simulink model "e1516sim"  (R2022a)
settings: Solver=VariableStepAuto  StartTime=0.0  StopTime=10  RelTol=1e-3
values from neighbouring files (symbols this model uses):
  delta_a = 0    [e1516.m]    (also in l6.m)
  dt = 0    [e1516.m]
  dy = 0    [e1516.m]
  rho = 1    [e1516.m]    (also in l6.m = 0)
libraries: cstblocks x2, simulink x1
settings Model: Creator=apple  LastModifiedBy=apple

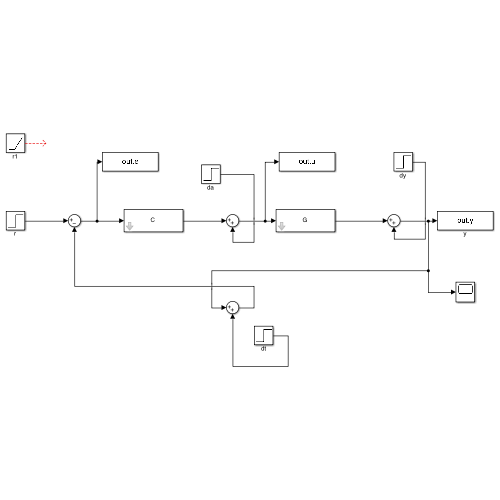
[thumbnail: Simulink's stored preview of the top-level diagram]
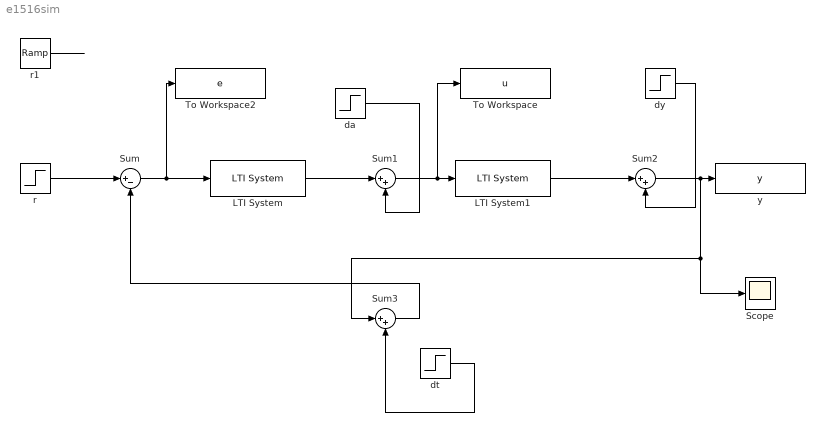
== system e1516sim ==
  LTI System : cstblocks/LTI System  sys=C  IC=[]
  LTI System1 : cstblocks/LTI System  sys=G  IC=[]
  Scope : Scope
  Sum : Sum  Inputs=|+-
  Sum1 : Sum  Inputs=|++
  Sum2 : Sum  Inputs=|++
  Sum3 : Sum  Inputs=|++
  To Workspace : ToWorkspace  VariableName=u  SaveFormat=Timeseries  SampleTime=-1
  To Workspace2 : ToWorkspace  VariableName=e  SaveFormat=Timeseries  SampleTime=-1
  da : Step  Time=0  After=delta_a  SampleTime=0
  dt : Step  Time=0  After=dt  SampleTime=0
  dy : Step  Time=0  After=dy  SampleTime=0
  r : Step  Time=0  After=rho  SampleTime=0
  r1 : simulink/Sources/Ramp  slope=rho  start=0  InitialOutput=0
  y : ToWorkspace  VariableName=y  SaveFormat=Timeseries  SampleTime=-1
  wires:
  dy/1 -> Sum2/2
  Sum2/1 -> Scope/1, Sum3/1, y/1
  dt/1 -> Sum3/2
  Sum3/1 -> Sum/2
  r/1 -> Sum/1
  Sum/1 -> To Workspace2/1, LTI System/1
  LTI System/1 -> Sum1/1
  Sum1/1 -> To Workspace/1, LTI System1/1
  da/1 -> Sum1/2
  LTI System1/1 -> Sum2/1
  r1/1 -> ?
